simulink model "PID_Error_test"  (R2024b)
settings: Solver=FixedStepAuto  StartTime=0.0  StopTime=1  FixedStep=0.1  RelTol=1e-3
settings Model: Creator=USER  LastModifiedBy=USER

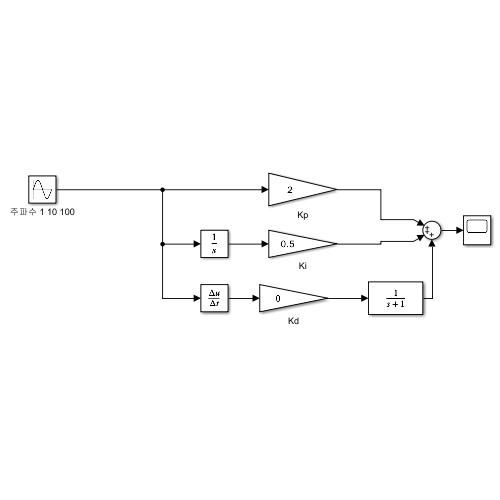
[thumbnail: Simulink's stored preview of the top-level diagram]
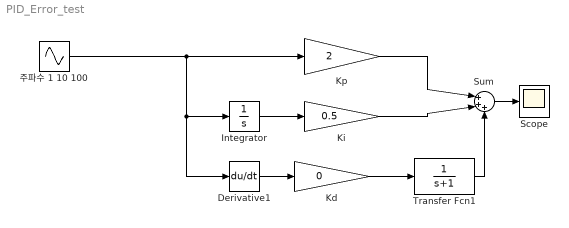
== system PID_Error_test ==
  Derivative1 : Derivative
  Integrator : Integrator
  Kd : Gain  Gain=0  ParamDataTypeStr=double  OutDataTypeStr=double
  Ki : Gain  Gain=0.5  ParamDataTypeStr=double  OutDataTypeStr=double
  Kp : Gain  Gain=2  ParamDataTypeStr=double  OutDataTypeStr=double
  Scope : Scope
  Sum : Sum  Inputs=|+++
  Transfer Fcn1 : TransferFcn  Denominator=[1 1]
  주파수 1 10 100 : Sin  Amplitude=150  Frequency=10  SampleTime=0
  wires:
  Integrator/1 -> Ki/1
  Kp/1 -> Sum/1
  Transfer Fcn1/1 -> Sum/3
  Ki/1 -> Sum/2
  주파수 1 10 100/1 -> Derivative1/1, Integrator/1, Kp/1
  Kd/1 -> Transfer Fcn1/1
  Derivative1/1 -> Kd/1
  Sum/1 -> Scope/1
